simulink model "capture"  (Simulink 7.0)
settings: Solver=ode45  StartTime=0.0  StopTime=100  RelTol=1e-3
libraries: xbsIndex_r4 x33, xps_library x6, isi_correlator_lib x2
settings Model: Creator=wjm  LastModifiedBy=wjm

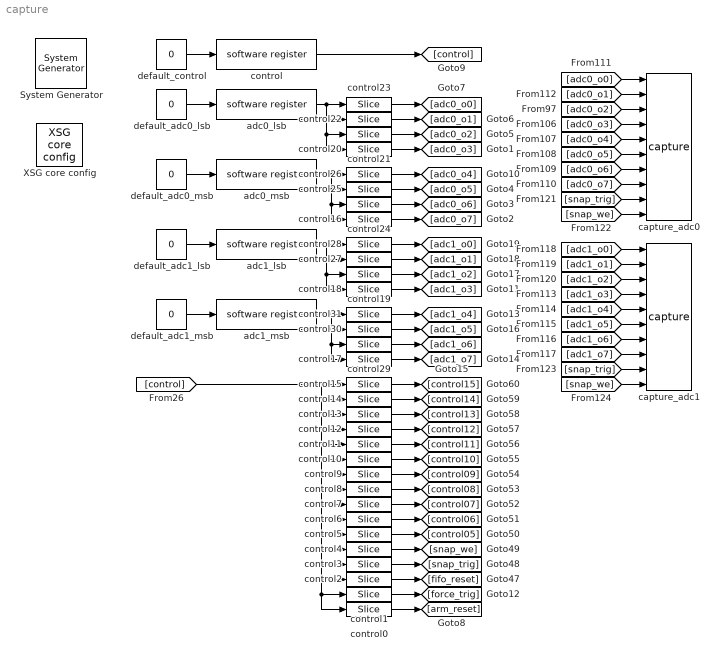
== system capture ==
  " System Generator" : xbsIndex_r4/ System Generator  Tag=genX  SystemSampleTime=-1  xilinxfamily=virtex5  part=xc5vsx95t  speed=-1  package=ff1136  synthesis_tool=XST  clock_wrapper=Clock Enables  directory=./capture/sysgen  testbench=off  simulink_period=1  sysclk_period=5  dcm_input_clock_period=100  incr_netlist=off  trim_vbits=Everywhere in SubSystem  dbl_ovrd=According to Block Masks  core_generation=According to Block Masks  run_coregen=off  deprecated_control=off  eval_field=0  block_type=sysgen
      settings: block_version=10.1.3
  XSG core config : xps_library/XSG core config  Tag=xps:xsg  SystemSampleTime=-1  hw_sys=ROACH:sx95t  ibob_linux=off  clk_src=sys_clk2x  iBOB_clk_src=sys_clk  BEE2_ctrl_clk_src=sys_clk  BEE2_usr_clk_src=sys_clk  ROACH_clk_src=sys_clk2x  CORR_clk_src=sys_clk  gpio_clk_io_group=iBOB:sma  gpio_clk_bit_index=0  clk_rate=200  sample_period=1  synthesis_tool=XST  mpc_type=powerpc440_ext
  adc0_lsb : xps_library/software register  Tag=xps:sw_reg  SystemSampleTime=-1  io_dir=From Processor  arith_type=Unsigned  bitwidth=32  bin_pt=0  sample_period=1  gw_name=capture_adc0_lsb_user_data_out
      link override capture_adc0_lsb_user_data_out: arith_type=Unsigned  n_bits=32  bin_pt=0  period=1
      link override corr_3ghz_10_1_corr_id_user_data_out: arith_type=Unsigned  n_bits=32  bin_pt=0  period=1
      link override corr_3ghz_10_1_exp_corr_id_user_data_out: arith_type=Unsigned  n_bits=32  bin_pt=0  period=1
      link override isi_corr_eq_coeff_user_data_out: arith_type=Unsigned  n_bits=32  bin_pt=0  period=1
      link override isi_correlator_control_user_data_out: arith_type=Unsigned  n_bits=32  bin_pt=0  period=1
      link override isi_correlator_cropped_control_user_data_out: arith_type=Unsigned  n_bits=32  bin_pt=0  period=1
      link override isi_correlator_eq_coeff_user_data_out: arith_type=Unsigned  n_bits=32  bin_pt=0  period=1
      link override untitled_adc0_lsb_user_data_out: arith_type=Unsigned  n_bits=32  bin_pt=0  period=1
  adc0_msb : xps_library/software register  Tag=xps:sw_reg  SystemSampleTime=-1  io_dir=From Processor  arith_type=Unsigned  bitwidth=32  bin_pt=0  sample_period=1  gw_name=capture_adc0_msb_user_data_out
      link override capture_adc0_msb_user_data_out: arith_type=Unsigned  n_bits=32  bin_pt=0  period=1
      link override corr_3ghz_10_1_corr_id_user_data_out: arith_type=Unsigned  n_bits=32  bin_pt=0  period=1
      link override corr_3ghz_10_1_exp_corr_id_user_data_out: arith_type=Unsigned  n_bits=32  bin_pt=0  period=1
      link override isi_corr_eq_coeff_user_data_out: arith_type=Unsigned  n_bits=32  bin_pt=0  period=1
      link override isi_correlator_control_user_data_out: arith_type=Unsigned  n_bits=32  bin_pt=0  period=1
      link override isi_correlator_cropped_control_user_data_out: arith_type=Unsigned  n_bits=32  bin_pt=0  period=1
      link override isi_correlator_eq_coeff_user_data_out: arith_type=Unsigned  n_bits=32  bin_pt=0  period=1
      link override untitled_adc0_msb_user_data_out: arith_type=Unsigned  n_bits=32  bin_pt=0  period=1
  adc1_lsb : xps_library/software register  Tag=xps:sw_reg  SystemSampleTime=-1  io_dir=From Processor  arith_type=Unsigned  bitwidth=32  bin_pt=0  sample_period=1  gw_name=capture_adc1_lsb_user_data_out
      link override capture_adc1_lsb_user_data_out: arith_type=Unsigned  n_bits=32  bin_pt=0  period=1
      link override corr_3ghz_10_1_corr_id_user_data_out: arith_type=Unsigned  n_bits=32  bin_pt=0  period=1
      link override corr_3ghz_10_1_exp_corr_id_user_data_out: arith_type=Unsigned  n_bits=32  bin_pt=0  period=1
      link override isi_corr_eq_coeff_user_data_out: arith_type=Unsigned  n_bits=32  bin_pt=0  period=1
      link override isi_correlator_control_user_data_out: arith_type=Unsigned  n_bits=32  bin_pt=0  period=1
      link override isi_correlator_cropped_control_user_data_out: arith_type=Unsigned  n_bits=32  bin_pt=0  period=1
      link override isi_correlator_eq_coeff_user_data_out: arith_type=Unsigned  n_bits=32  bin_pt=0  period=1
      link override untitled_adc1_lsb_user_data_out: arith_type=Unsigned  n_bits=32  bin_pt=0  period=1
  adc1_msb : xps_library/software register  Tag=xps:sw_reg  SystemSampleTime=-1  io_dir=From Processor  arith_type=Unsigned  bitwidth=32  bin_pt=0  sample_period=1  gw_name=capture_adc1_msb_user_data_out
      link override capture_adc1_msb_user_data_out: arith_type=Unsigned  n_bits=32  bin_pt=0  period=1
      link override corr_3ghz_10_1_corr_id_user_data_out: arith_type=Unsigned  n_bits=32  bin_pt=0  period=1
      link override corr_3ghz_10_1_exp_corr_id_user_data_out: arith_type=Unsigned  n_bits=32  bin_pt=0  period=1
      link override isi_corr_eq_coeff_user_data_out: arith_type=Unsigned  n_bits=32  bin_pt=0  period=1
      link override isi_correlator_control_user_data_out: arith_type=Unsigned  n_bits=32  bin_pt=0  period=1
      link override isi_correlator_cropped_control_user_data_out: arith_type=Unsigned  n_bits=32  bin_pt=0  period=1
      link override isi_correlator_eq_coeff_user_data_out: arith_type=Unsigned  n_bits=32  bin_pt=0  period=1
      link override untitled_adc1_msb_user_data_out: arith_type=Unsigned  n_bits=32  bin_pt=0  period=1
  capture_adc0 : isi_correlator_lib/capture  SystemSampleTime=-1
      link override snap64/addr/convert: arith_type=Unsigned  n_bits=32  bin_pt=0
      link override snap64/bram_lsb/capture_capture_adc0_snap64_bram_lsb_data_out: arith_type=Unsigned
      link override snap64/bram_lsb/convert_din: arith_type=Unsigned
      link override snap64/bram_lsb/isi_correlator_capture_adc0_snap64_bram_lsb_data_out: arith_type=Unsigned
      link override snap64/bram_lsb/mem/sim_data_in: arith_type=Unsigned
      link override snap64/bram_lsb/untitled_capture_adc0_snap64_bram_lsb_data_out: arith_type=Unsigned
      link override snap64/bram_msb/capture_capture_adc0_snap64_bram_msb_data_out: arith_type=Unsigned
      link override snap64/bram_msb/convert_din: arith_type=Unsigned
      link override snap64/bram_msb/isi_correlator_capture_adc0_snap64_bram_msb_data_out: arith_type=Unsigned
      link override snap64/bram_msb/mem/sim_data_in: arith_type=Unsigned
      link override snap64/bram_msb/untitled_capture_adc0_snap64_bram_msb_data_out: arith_type=Unsigned
      link override snap64/ctrl/capture_capture_adc0_snap64_ctrl_user_data_out: arith_type=Unsigned  n_bits=32  bin_pt=0  period=1
      link override snap64/ctrl/isi_correlator_capture_adc0_snap64_ctrl_user_data_out: arith_type=Unsigned  n_bits=32  bin_pt=0  period=1
      link override snap64/ctrl/untitled_capture_adc0_snap64_ctrl_user_data_out: arith_type=Unsigned  n_bits=32  bin_pt=0  period=1
  capture_adc1 : isi_correlator_lib/capture  SystemSampleTime=-1
      link override snap64/addr/convert: arith_type=Unsigned  n_bits=32  bin_pt=0
      link override snap64/bram_lsb/capture_capture_adc1_snap64_bram_lsb_data_out: arith_type=Unsigned
      link override snap64/bram_lsb/convert_din: arith_type=Unsigned
      link override snap64/bram_lsb/isi_correlator_capture_adc1_snap64_bram_lsb_data_out: arith_type=Unsigned
      link override snap64/bram_lsb/mem/sim_data_in: arith_type=Unsigned
      link override snap64/bram_lsb/untitled_capture_adc1_snap64_bram_lsb_data_out: arith_type=Unsigned
      link override snap64/bram_msb/capture_capture_adc1_snap64_bram_msb_data_out: arith_type=Unsigned
      link override snap64/bram_msb/convert_din: arith_type=Unsigned
      link override snap64/bram_msb/isi_correlator_capture_adc1_snap64_bram_msb_data_out: arith_type=Unsigned
      link override snap64/bram_msb/mem/sim_data_in: arith_type=Unsigned
      link override snap64/bram_msb/untitled_capture_adc1_snap64_bram_msb_data_out: arith_type=Unsigned
      link override snap64/ctrl/capture_capture_adc1_snap64_ctrl_user_data_out: arith_type=Unsigned  n_bits=32  bin_pt=0  period=1
      link override snap64/ctrl/isi_correlator_capture_adc1_snap64_ctrl_user_data_out: arith_type=Unsigned  n_bits=32  bin_pt=0  period=1
      link override snap64/ctrl/untitled_capture_adc1_snap64_ctrl_user_data_out: arith_type=Unsigned  n_bits=32  bin_pt=0  period=1
  control : xps_library/software register  Tag=xps:sw_reg  SystemSampleTime=-1  io_dir=From Processor  arith_type=Unsigned  bitwidth=32  bin_pt=0  sample_period=1  gw_name=capture_control_user_data_out
      link override capture_control_user_data_out: arith_type=Unsigned  n_bits=32  bin_pt=0  period=1
      link override corr_3ghz_10_1_corr_id_user_data_out: arith_type=Unsigned  n_bits=32  bin_pt=0  period=1
      link override corr_3ghz_10_1_exp_corr_id_user_data_out: arith_type=Unsigned  n_bits=32  bin_pt=0  period=1
      link override isi_corr_eq_coeff_user_data_out: arith_type=Unsigned  n_bits=32  bin_pt=0  period=1
      link override isi_correlator_control_user_data_out: arith_type=Unsigned  n_bits=32  bin_pt=0  period=1
      link override isi_correlator_cropped_control_user_data_out: arith_type=Unsigned  n_bits=32  bin_pt=0  period=1
      link override isi_correlator_eq_coeff_user_data_out: arith_type=Unsigned  n_bits=32  bin_pt=0  period=1
      link override untitled_control_user_data_out: arith_type=Unsigned  n_bits=32  bin_pt=0  period=1
  control0 : xbsIndex_r4/Slice  nbits=1  boolean_output=on  mode=Lower Bit Location + Width  bit1=0  base1=MSB of Input  bit0=0  base0=LSB of Input  dbl_ovrd=off  block_type=slice
      settings: infoedit="Extracts a given range of bits from each input sample and presents it at the output.  The output type is ordinarily unsigned with binary point at zero, but can be Boolean when the slice is one bit wide.<P><P>Hardware notes: In hardware this block costs nothing."  block_version=10.1.3
  control1 : xbsIndex_r4/Slice  nbits=1  boolean_output=on  mode=Lower Bit Location + Width  bit1=0  base1=MSB of Input  bit0=1  base0=LSB of Input  dbl_ovrd=off  block_type=slice
      settings: infoedit="Extracts a given range of bits from each input sample and presents it at the output.  The output type is ordinarily unsigned with binary point at zero, but can be Boolean when the slice is one bit wide.<P><P>Hardware notes: In hardware this block costs nothing."  block_version=10.1.3
  control10 : xbsIndex_r4/Slice  nbits=1  boolean_output=on  mode=Lower Bit Location + Width  bit1=0  base1=MSB of Input  bit0=10  base0=LSB of Input  dbl_ovrd=off  block_type=slice
      settings: infoedit="Extracts a given range of bits from each input sample and presents it at the output.  The output type is ordinarily unsigned with binary point at zero, but can be Boolean when the slice is one bit wide.<P><P>Hardware notes: In hardware this block costs nothing."  block_version=10.1.3
  control11 : xbsIndex_r4/Slice  nbits=1  boolean_output=on  mode=Lower Bit Location + Width  bit1=0  base1=MSB of Input  bit0=11  base0=LSB of Input  dbl_ovrd=off  block_type=slice
      settings: infoedit="Extracts a given range of bits from each input sample and presents it at the output.  The output type is ordinarily unsigned with binary point at zero, but can be Boolean when the slice is one bit wide.<P><P>Hardware notes: In hardware this block costs nothing."  block_version=10.1.3
  control12 : xbsIndex_r4/Slice  nbits=1  boolean_output=on  mode=Lower Bit Location + Width  bit1=0  base1=MSB of Input  bit0=12  base0=LSB of Input  dbl_ovrd=off  block_type=slice
      settings: infoedit="Extracts a given range of bits from each input sample and presents it at the output.  The output type is ordinarily unsigned with binary point at zero, but can be Boolean when the slice is one bit wide.<P><P>Hardware notes: In hardware this block costs nothing."  block_version=10.1.3
  control13 : xbsIndex_r4/Slice  nbits=1  boolean_output=on  mode=Lower Bit Location + Width  bit1=0  base1=MSB of Input  bit0=13  base0=LSB of Input  dbl_ovrd=off  block_type=slice
      settings: infoedit="Extracts a given range of bits from each input sample and presents it at the output.  The output type is ordinarily unsigned with binary point at zero, but can be Boolean when the slice is one bit wide.<P><P>Hardware notes: In hardware this block costs nothing."  block_version=10.1.3
  control14 : xbsIndex_r4/Slice  nbits=1  boolean_output=on  mode=Lower Bit Location + Width  bit1=0  base1=MSB of Input  bit0=14  base0=LSB of Input  dbl_ovrd=off  block_type=slice
      settings: infoedit="Extracts a given range of bits from each input sample and presents it at the output.  The output type is ordinarily unsigned with binary point at zero, but can be Boolean when the slice is one bit wide.<P><P>Hardware notes: In hardware this block costs nothing."  block_version=10.1.3
  control15 : xbsIndex_r4/Slice  nbits=1  boolean_output=on  mode=Lower Bit Location + Width  bit1=0  base1=MSB of Input  bit0=15  base0=LSB of Input  dbl_ovrd=off  block_type=slice
      settings: infoedit="Extracts a given range of bits from each input sample and presents it at the output.  The output type is ordinarily unsigned with binary point at zero, but can be Boolean when the slice is one bit wide.<P><P>Hardware notes: In hardware this block costs nothing."  block_version=10.1.3
  control{16..18,20} (4 alike) : xbsIndex_r4/Slice  nbits=8  boolean_output=off  mode=Lower Bit Location + Width  bit1=0  base1=MSB of Input  bit0=24  base0=LSB of Input  dbl_ovrd=off  block_type=slice
      settings: infoedit="Extracts a given range of bits from each input sample and presents it at the output.  The output type is ordinarily unsigned with binary point at zero, but can be Boolean when the slice is one bit wide.<P><P>Hardware notes: In hardware this block costs nothing."  block_version=10.1.3
  control{19,21,24,29} (4 alike) : xbsIndex_r4/Slice  nbits=8  boolean_output=off  mode=Lower Bit Location + Width  bit1=0  base1=MSB of Input  bit0=16  base0=LSB of Input  dbl_ovrd=off  block_type=slice
      settings: infoedit="Extracts a given range of bits from each input sample and presents it at the output.  The output type is ordinarily unsigned with binary point at zero, but can be Boolean when the slice is one bit wide.<P><P>Hardware notes: In hardware this block costs nothing."  block_version=10.1.3
  control2 : xbsIndex_r4/Slice  nbits=1  boolean_output=on  mode=Lower Bit Location + Width  bit1=0  base1=MSB of Input  bit0=2  base0=LSB of Input  dbl_ovrd=off  block_type=slice
      settings: infoedit="Extracts a given range of bits from each input sample and presents it at the output.  The output type is ordinarily unsigned with binary point at zero, but can be Boolean when the slice is one bit wide.<P><P>Hardware notes: In hardware this block costs nothing."  block_version=10.1.3
  control{22,25,27,30} (4 alike) : xbsIndex_r4/Slice  nbits=8  boolean_output=off  mode=Lower Bit Location + Width  bit1=0  base1=MSB of Input  bit0=8  base0=LSB of Input  dbl_ovrd=off  block_type=slice
      settings: infoedit="Extracts a given range of bits from each input sample and presents it at the output.  The output type is ordinarily unsigned with binary point at zero, but can be Boolean when the slice is one bit wide.<P><P>Hardware notes: In hardware this block costs nothing."  block_version=10.1.3
  control{23,26,28,31} (4 alike) : xbsIndex_r4/Slice  nbits=8  boolean_output=off  mode=Lower Bit Location + Width  bit1=0  base1=MSB of Input  bit0=0  base0=LSB of Input  dbl_ovrd=off  block_type=slice
      settings: infoedit="Extracts a given range of bits from each input sample and presents it at the output.  The output type is ordinarily unsigned with binary point at zero, but can be Boolean when the slice is one bit wide.<P><P>Hardware notes: In hardware this block costs nothing."  block_version=10.1.3
  control3 : xbsIndex_r4/Slice  nbits=1  boolean_output=on  mode=Lower Bit Location + Width  bit1=0  base1=MSB of Input  bit0=3  base0=LSB of Input  dbl_ovrd=off  block_type=slice
      settings: infoedit="Extracts a given range of bits from each input sample and presents it at the output.  The output type is ordinarily unsigned with binary point at zero, but can be Boolean when the slice is one bit wide.<P><P>Hardware notes: In hardware this block costs nothing."  block_version=10.1.3
  control4 : xbsIndex_r4/Slice  nbits=1  boolean_output=on  mode=Lower Bit Location + Width  bit1=0  base1=MSB of Input  bit0=4  base0=LSB of Input  dbl_ovrd=off  block_type=slice
      settings: infoedit="Extracts a given range of bits from each input sample and presents it at the output.  The output type is ordinarily unsigned with binary point at zero, but can be Boolean when the slice is one bit wide.<P><P>Hardware notes: In hardware this block costs nothing."  block_version=10.1.3
  control5 : xbsIndex_r4/Slice  nbits=1  boolean_output=on  mode=Lower Bit Location + Width  bit1=0  base1=MSB of Input  bit0=5  base0=LSB of Input  dbl_ovrd=off  block_type=slice
      settings: infoedit="Extracts a given range of bits from each input sample and presents it at the output.  The output type is ordinarily unsigned with binary point at zero, but can be Boolean when the slice is one bit wide.<P><P>Hardware notes: In hardware this block costs nothing."  block_version=10.1.3
  control6 : xbsIndex_r4/Slice  nbits=1  boolean_output=on  mode=Lower Bit Location + Width  bit1=0  base1=MSB of Input  bit0=6  base0=LSB of Input  dbl_ovrd=off  block_type=slice
      settings: infoedit="Extracts a given range of bits from each input sample and presents it at the output.  The output type is ordinarily unsigned with binary point at zero, but can be Boolean when the slice is one bit wide.<P><P>Hardware notes: In hardware this block costs nothing."  block_version=10.1.3
  control7 : xbsIndex_r4/Slice  nbits=1  boolean_output=on  mode=Lower Bit Location + Width  bit1=0  base1=MSB of Input  bit0=7  base0=LSB of Input  dbl_ovrd=off  block_type=slice
      settings: infoedit="Extracts a given range of bits from each input sample and presents it at the output.  The output type is ordinarily unsigned with binary point at zero, but can be Boolean when the slice is one bit wide.<P><P>Hardware notes: In hardware this block costs nothing."  block_version=10.1.3
  control8 : xbsIndex_r4/Slice  nbits=1  boolean_output=on  mode=Lower Bit Location + Width  bit1=0  base1=MSB of Input  bit0=8  base0=LSB of Input  dbl_ovrd=off  block_type=slice
      settings: infoedit="Extracts a given range of bits from each input sample and presents it at the output.  The output type is ordinarily unsigned with binary point at zero, but can be Boolean when the slice is one bit wide.<P><P>Hardware notes: In hardware this block costs nothing."  block_version=10.1.3
  control9 : xbsIndex_r4/Slice  nbits=1  boolean_output=on  mode=Lower Bit Location + Width  bit1=0  base1=MSB of Input  bit0=9  base0=LSB of Input  dbl_ovrd=off  block_type=slice
      settings: infoedit="Extracts a given range of bits from each input sample and presents it at the output.  The output type is ordinarily unsigned with binary point at zero, but can be Boolean when the slice is one bit wide.<P><P>Hardware notes: In hardware this block costs nothing."  block_version=10.1.3
  default_adc0_lsb : Constant  Value=0  OutDataType=sfix(16)  OutScaling=2^0  SampleTime=1
  default_adc0_msb : Constant  Value=0  OutDataType=sfix(16)  OutScaling=2^0  SampleTime=1
  default_adc1_lsb : Constant  Value=0  OutDataType=sfix(16)  OutScaling=2^0  SampleTime=1
  default_adc1_msb : Constant  Value=0  OutDataType=sfix(16)  OutScaling=2^0  SampleTime=1
  default_control : Constant  Value=0  OutDataType=sfix(16)  OutScaling=2^0  SampleTime=1
  wires:
  [adc0_o0] -> capture_adc0/1
  [adc0_o1] -> capture_adc0/2
  [adc0_o2] -> capture_adc0/3
  [adc0_o3] -> capture_adc0/4
  [adc0_o4] -> capture_adc0/5
  [adc0_o5] -> capture_adc0/6
  [adc0_o6] -> capture_adc0/7
  [adc0_o7] -> capture_adc0/8
  [adc1_o0] -> capture_adc1/1
  [adc1_o1] -> capture_adc1/2
  [adc1_o2] -> capture_adc1/3
  [adc1_o3] -> capture_adc1/4
  [adc1_o4] -> capture_adc1/5
  [adc1_o5] -> capture_adc1/6
  [adc1_o6] -> capture_adc1/7
  [adc1_o7] -> capture_adc1/8
  [snap_trig] -> capture_adc0/9
  [snap_we] -> capture_adc0/10
  [snap_trig] -> capture_adc1/9
  [snap_we] -> capture_adc1/10
  default_control/1 -> control/1
  control/1 -> [control]
  [control] -> control15/1, control14/1, control13/1, control12/1, control11/1, control10/1, control9/1, control8/1, control7/1, control6/1, control5/1, control4/1, control3/1, control2/1, control1/1, control0/1
  control15/1 -> [control15]
  control14/1 -> [control14]
  control13/1 -> [control13]
  control12/1 -> [control12]
  control11/1 -> [control11]
  control10/1 -> [control10]
  control9/1 -> [control09]
  control8/1 -> [control08]
  control7/1 -> [control07]
  control6/1 -> [control06]
  control5/1 -> [control05]
  control4/1 -> [snap_we]
  control3/1 -> [snap_trig]
  control2/1 -> [fifo_reset]
  control1/1 -> [force_trig]
  control0/1 -> [arm_reset]
  control23/1 -> [adc0_o0]
  control22/1 -> [adc0_o1]
  control21/1 -> [adc0_o2]
  control20/1 -> [adc0_o3]
  adc0_lsb/1 -> control23/1, control22/1, control21/1, control20/1
  control26/1 -> [adc0_o4]
  control25/1 -> [adc0_o5]
  control24/1 -> [adc0_o6]
  control16/1 -> [adc0_o7]
  adc0_msb/1 -> control26/1, control25/1, control24/1, control16/1
  default_adc0_lsb/1 -> adc0_lsb/1
  default_adc0_msb/1 -> adc0_msb/1
  control28/1 -> [adc1_o0]
  control27/1 -> [adc1_o1]
  control19/1 -> [adc1_o2]
  control18/1 -> [adc1_o3]
  adc1_lsb/1 -> control28/1, control27/1, control19/1, control18/1
  control31/1 -> [adc1_o4]
  control30/1 -> [adc1_o5]
  control29/1 -> [adc1_o6]
  control17/1 -> [adc1_o7]
  adc1_msb/1 -> control31/1, control30/1, control29/1, control17/1
  default_adc1_lsb/1 -> adc1_lsb/1
  default_adc1_msb/1 -> adc1_msb/1
